simulink model "screening_workflow"  (R2026a)
settings: Solver=ode23tb  StopTime=2400
PreLoadFcn:
  | P = screening_params();
InitFcn:
  | P = screening_params();
settings Model: Creator=dines  LastModifiedBy=dines

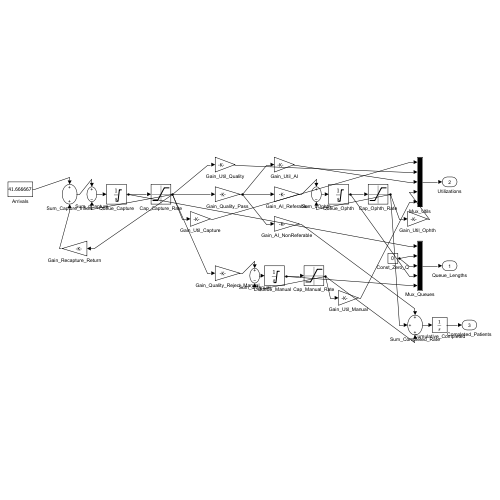
[thumbnail: Simulink's stored preview of the top-level diagram]
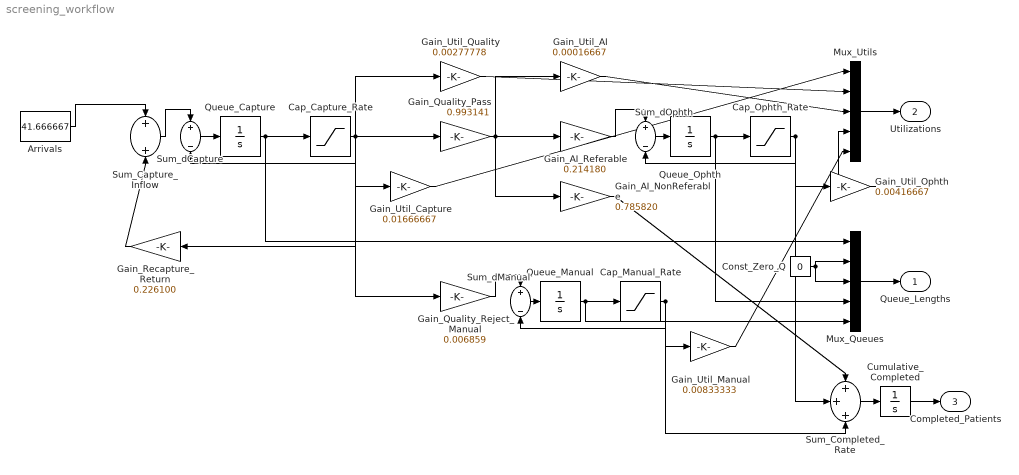
== system screening_workflow ==
  Arrivals : Constant  Value=41.666667
  Cap_Capture_Rate : Saturate  UpperLimit=60.000000  LowerLimit=0
  Cap_Manual_Rate : Saturate  UpperLimit=120.000000  LowerLimit=0
  Cap_Ophth_Rate : Saturate  UpperLimit=240.000000  LowerLimit=0
  Const_Zero_Q : Constant  Value=0
  Cumulative_Completed : Integrator
  Gain_AI_NonReferable : Gain  Gain=0.785820
  Gain_AI_Referable : Gain  Gain=0.214180
  Gain_Quality_Pass : Gain  Gain=0.993141
  Gain_Quality_Reject_Manual : Gain  Gain=0.006859
  Gain_Recapture_Return : Gain  Gain=0.226100
  Gain_Util_AI : Gain  Gain=0.00016667
  Gain_Util_Capture : Gain  Gain=0.01666667
  Gain_Util_Manual : Gain  Gain=0.00833333
  Gain_Util_Ophth : Gain  Gain=0.00416667
  Gain_Util_Quality : Gain  Gain=0.00277778
  Mux_Queues : Mux  Inputs=5
  Mux_Utils : Mux  Inputs=5
  Queue_Capture : Integrator  LimitOutput=on  LowerSaturationLimit=0
  Queue_Manual : Integrator  LimitOutput=on  LowerSaturationLimit=0
  Queue_Ophth : Integrator  LimitOutput=on  LowerSaturationLimit=0
  Sum_Capture_Inflow : Sum
  Sum_Completed_Rate : Sum  Inputs=+++
  Sum_dCapture : Sum  Inputs=+-
  Sum_dManual : Sum  Inputs=+-
  Sum_dOphth : Sum  Inputs=+-
  Queue_Lengths : Outport
  Utilizations : Outport  Port=2
  Completed_Patients : Outport  Port=3
  wires:
  Arrivals/1 -> Sum_Capture_Inflow/1
  Gain_Recapture_Return/1 -> Sum_Capture_Inflow/2
  Sum_Capture_Inflow/1 -> Sum_dCapture/1
  Sum_dCapture/1 -> Queue_Capture/1
  Queue_Capture/1 -> Cap_Capture_Rate/1, Mux_Queues/1
  Cap_Capture_Rate/1 -> Sum_dCapture/2, Gain_Util_Capture/1, Gain_Recapture_Return/1, Gain_Quality_Pass/1, Gain_Quality_Reject_Manual/1, Gain_Util_Quality/1
  Gain_Quality_Pass/1 -> Gain_AI_Referable/1, Gain_AI_NonReferable/1, Gain_Util_AI/1
  Gain_AI_Referable/1 -> Sum_dOphth/1
  Sum_dOphth/1 -> Queue_Ophth/1
  Queue_Ophth/1 -> Cap_Ophth_Rate/1, Mux_Queues/4
  Cap_Ophth_Rate/1 -> Sum_dOphth/2, Gain_Util_Ophth/1, Sum_Completed_Rate/2
  Gain_Quality_Reject_Manual/1 -> Sum_dManual/1
  Sum_dManual/1 -> Queue_Manual/1
  Queue_Manual/1 -> Cap_Manual_Rate/1, Mux_Queues/5
  Cap_Manual_Rate/1 -> Sum_dManual/2, Gain_Util_Manual/1, Sum_Completed_Rate/3
  Gain_Util_Capture/1 -> Mux_Utils/1
  Gain_Util_Quality/1 -> Mux_Utils/2
  Gain_Util_AI/1 -> Mux_Utils/3
  Gain_Util_Ophth/1 -> Mux_Utils/4
  Gain_Util_Manual/1 -> Mux_Utils/5
  Mux_Utils/1 -> Utilizations/1
  Const_Zero_Q/1 -> Mux_Queues/2, Mux_Queues/3
  Mux_Queues/1 -> Queue_Lengths/1
  Gain_AI_NonReferable/1 -> Sum_Completed_Rate/1
  Sum_Completed_Rate/1 -> Cumulative_Completed/1
  Cumulative_Completed/1 -> Completed_Patients/1
